simulink model "hw2_Q1"  (R2022b)
settings: Solver=VariableStepAuto  StartTime=0.0  StopTime=5  RelTol=1e-3
libraries: simulink x1
settings Model: Creator=morteza  LastModifiedBy=shivavafadar
settings SolverCC: AlgebraicLoopSolver=TrustRegion
settings DebuggingCC: UnconnectedInputMsg=warning  UnconnectedOutputMsg=warning  UnconnectedLineMsg=warning  SFMachineParentedDataDiag=warning
settings ModelReferenceCC: EnableRefExpFcnMdlSchedulingChecks=on
settings RTWCC: DLArmComputeVersion=19.05

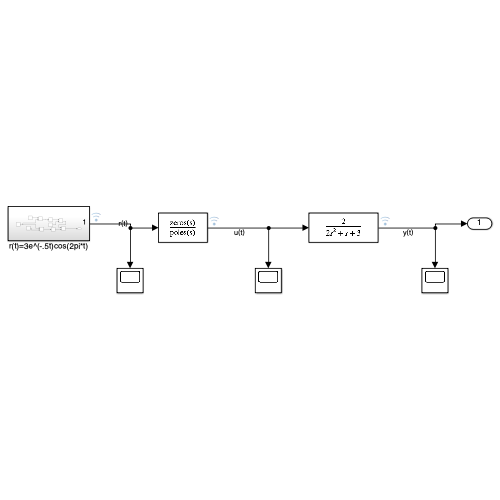
[thumbnail: Simulink's stored preview of the top-level diagram]
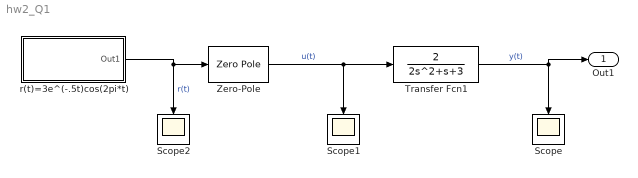
== system hw2_Q1 ==
  Scope : Scope
  Scope1 : Scope
  Scope2 : Scope
  Transfer Fcn1 : TransferFcn  Numerator=[2]  Denominator=[2,1,3]
  Zero-Pole : ZeroPole  Zeros=[-4]  Poles=[0 -1]
  r(t)=3e^(-.5t)cos(2pi*t) : Subsystem
  Out1 : Outport
  wires:
  Zero-Pole/1 -> Transfer Fcn1/1, Scope1/1  "u(t)"
  r(t)=3e^(-.5t)cos(2pi*t)/1(Out1) -> Zero-Pole/1, Scope2/1  "r(t)"
  Transfer Fcn1/1 -> Out1/1, Scope/1  "y(t)"

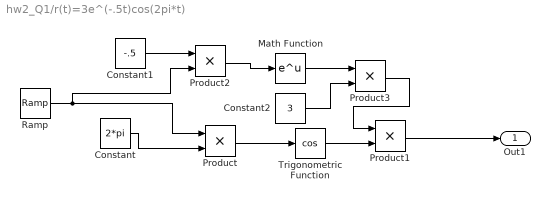
== system hw2_Q1/r(t)=3e^(-.5t)cos(2pi*t) ==
  Constant : Constant  Value=2*pi
  Constant1 : Constant  Value=-.5
  Constant2 : Constant  Value=3
  Math Function : Math
  Product{,1..3} (4 alike) : Product
  Ramp : simulink/Sources/Ramp  slope=1  start=0  InitialOutput=0
  Trigonometric Function : Trigonometry  Operator=cos
  Out1 : Outport
  wires:
  Product2/1 -> Math Function/1
  Trigonometric Function/1 -> Product1/2
  Product/1 -> Trigonometric Function/1
  Math Function/1 -> Product3/1
  Constant2/1 -> Product3/2
  Product3/1 -> Product1/1
  Constant1/1 -> Product2/1
  Ramp/1 -> Product2/2, Product/1
  Constant/1 -> Product/2
  Product1/1 -> Out1/1
